simulink model "inpguitest"  (Simulink 9.1)
settings: Solver=FixedStepDiscrete  StartTime=0.0  StopTime=inf  RelTol=1e-3  EnableMultiTasking=on
libraries: fuzblock x1
settings Model: Creator=nskandan  LastModifiedBy=PC
settings DataIOCC: LimitDataPoints=on  SignalLoggingSaveFormat=ModelDataLogs
settings OptimizationCC: InitFltsAndDblsToZero=on
settings DebuggingCC: SaveWithParameterizedLinksMsg=none  SignalResolutionControl=TryResolveAllWithWarning  SolverPrmCheckMsg=warning  FcnCallInpInsideContextMsg=warning
settings GRTTargetCC: TargetFcnLib=ansi_tfl_tmw.mat

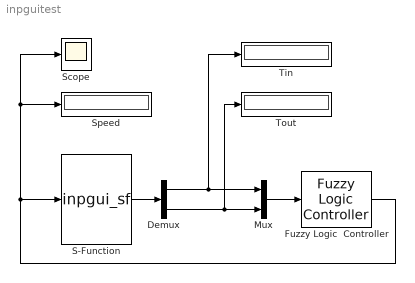
== system inpguitest ==
  Demux : Demux  Outputs=2
  Fuzzy Logic  Controller : fuzblock/Fuzzy Logic  Controller  FIS='fuzzy_2in_1out.fis'  OutputSampleNumber=101  DataType=double  FuzzifiedInputs=off  RuleFiringStrengths=off  RuleOutputs=off  AggregatedOutputs=off  SimulateUsing=Interpreted execution  OutOfRangeInputValueMessage=warning  NoRuleFiredMessage=warning  EmptyOutputFuzzySetMessage=warning
  Mux : Mux  Inputs=2
  S-Function : S-Function  FunctionName=inpgui_sf  Parameters=0.005  SFunctionDeploymentMode=off  EnableBusSupport=off
  Scope : Scope
  "Speed " : Display
  "Tin  " : Display
  "Tout  " : Display
  wires:
  S-Function/1 -> Demux/1
  Mux/1 -> Fuzzy Logic  Controller/1
  Demux/1 -> Mux/1, "Tin  "/1
  Fuzzy Logic  Controller/1 -> Scope/1, "Speed "/1, S-Function/1
  Demux/2 -> "Tout  "/1, Mux/2
